simulink model "inverseDynamicsControl"  (R2023b)
settings: Solver=VariableStepAuto  StartTime=0.0  StopTime=time(end)  RelTol=1e-3
undefined symbols (not defined in the file): DiscIntNeverNeededParam
libraries: simulink x1, slpidlib x1
settings Model: Creator=v4pal  LastModifiedBy=v4pal

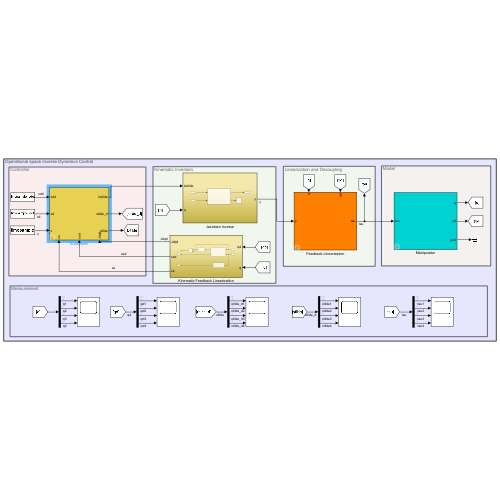
[thumbnail: Simulink's stored preview of the top-level diagram]
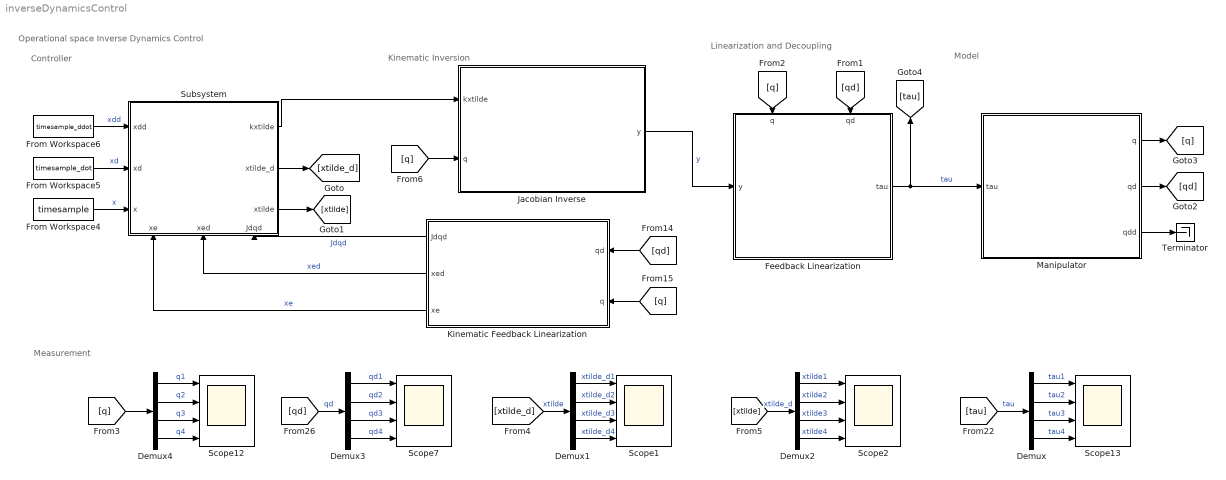
== system inverseDynamicsControl ==
  note: Measurement
  note: Operational space Inverse Dynamics Control
  note: Controller
  note: Kinematic Inversion
  note: Model
  note: Linearization and Decoupling
  Demux{,1..4} (5 alike) : Demux
  Feedback Linearization : Subsystem  mask{m_load=4}
      mask prompts: m_load "Load Mass [kg]"
      settings: PortSchema="{\"entries\":[{\"content\":{\"sides\":[{\"content\":{\"connectorIds\":[\"In1\"]},\"type\":\"ConnectorPlacement.EquallySpacedRectSide\",\"uuid\":\"271cc0a6-b732-4626-ad15-944ba501bea2\"},{\"content\":{\"connectorIds\":[\"Out1\"],\"side\":\"RIGHT\"},\"type\":\"ConnectorPlacement.EquallySpacedRectSide\",\"uuid\":\"860ec51b-c9e7-4b7b-ae65-2fc3300d48f6\"},{\"content\":{\"connectorIds\":[\"In2\",\"In3\"],\"side\":\"TOP\"},\"type\":\"ConnectorPlacement.EquallySpacedRectSide\",\"uuid\":\"a378ade9-13de-47ec-a220-3e435cc4dc56\"},{\"content\":{\"side\":\"BOTTOM\"},\"type\":\"ConnectorPlacement.EquallySpacedRectSide\",\"uuid\":\"8c63b252-3c1f-48d2-9139-67a3c74d1549\"}]},\"type\":\"ConnectorPlacement.EquallySpacedConnector\",\"uuid\":\"fa57dee9-db69-4719-bb64-b991f88f74fb\"}],\"packageUris\":[\"http://schema.mathworks.com/mf0/Connector/R2020b\"],\"version\":\"1.0\"}"
      mask DialogControl DescGroupVar Prompt: Nonlinear Compensation
      mask DialogControl DescTextVar Prompt: Nonlinear compensation and decoupling block
  From Workspace4 : FromWorkspace  VariableName=timesample
  From Workspace5 : FromWorkspace  VariableName=timesample_dot
  From Workspace6 : FromWorkspace  VariableName=timesample_ddot
  Jacobian Inverse : Subsystem
  Kinematic Feedback Linearization : Subsystem
  Manipulator : Subsystem  mask{m_load=4, delta=0.0}
      mask prompts: m_load "Load Mass [kg]"; delta "Uncertainty [%]"
      mask DialogControl DescGroupVar Prompt: SCARA Dynamic Model
      mask DialogControl DescTextVar Prompt: Scara Dynamic Model with uncertainty and load mass as input.
  Scope{1..2,7,12..13} (5 alike) : Scope  NumInputPorts=4
  Subsystem : Subsystem  mask{Kd=15, Kp=150, Ki=0}
      settings: PortSchema="{\"entries\":[{\"content\":{\"sides\":[{\"content\":{\"connectorIds\":[\"In1\",\"In2\",\"In3\"]},\"type\":\"ConnectorPlacement.EquallySpacedRectSide\",\"uuid\":\"d5d0fa15-0dfc-4de5-8b58-3094a24c3543\"},{\"content\":{\"connectorIds\":[\"Out1\",\"Out2\",\"Out3\"],\"side\":\"RIGHT\"},\"type\":\"ConnectorPlacement.EquallySpacedRectSide\",\"uuid\":\"dc48d10e-f543-4bb1-aabf-9e7d159af175\"},{\"content\":{\"side\":\"TOP\"},\"type\":\"ConnectorPlacement.EquallySpacedRectSide\",\"uuid\":\"cd48e311-8a6b-415c-be96-943e62210695\"},{\"content\":{\"connectorIds\":[\"In4\",\"In5\",\"In6\"],\"side\":\"BOTTOM\"},\"type\":\"ConnectorPlacement.EquallySpacedRectSide\",\"uuid\":\"938f084a-ffdf-47d0-9ea2-b90851473a83\"}]},\"type\":\"ConnectorPlacement.EquallySpacedConnector\",\"uuid\":\"fa3c2d25-ad58-4bec-8aba-e67d02255a63\"}],\"packageUris\":[\"http://schema.mathworks.com/mf0/Connector/R2020b\"],\"version\":\"1.0\"}"
  Terminator : Terminator
  wires:
  [qd] -> Kinematic Feedback Linearization/1(qd)
  [q] -> Kinematic Feedback Linearization/2(q)
  Feedback Linearization/1(tau) -> Manipulator/1(tau), [tau]  "tau"
  [qd] -> Feedback Linearization/3(qd)
  [q] -> Feedback Linearization/2(q)
  Manipulator/3(qdd) -> Terminator/1
  From Workspace6/1 -> Subsystem/1(xdd)  "xdd"
  From Workspace5/1 -> Subsystem/2(xd)  "xd"
  From Workspace4/1 -> Subsystem/3(x)  "x"
  Kinematic Feedback Linearization/1(Jdqd) -> Subsystem/6(Jdqd)  "Jdqd"
  Kinematic Feedback Linearization/2(xed) -> Subsystem/5(xed)  "xed"
  Kinematic Feedback Linearization/3(xe) -> Subsystem/4(xe)  "xe"
  Subsystem/1(kxtilde) -> Jacobian Inverse/1(kxtilde)
  Subsystem/2(xtilde_d) -> [xtilde_d]
  Subsystem/3(xtilde) -> [xtilde]
  Demux2/4 -> Scope2/4  "xtilde4"
  Demux2/3 -> Scope2/3  "xtilde3"
  Demux2/2 -> Scope2/2  "xtilde2"
  Demux2/1 -> Scope2/1  "xtilde1"
  Demux/2 -> Scope13/2  "tau2"
  Demux3/1 -> Scope7/1  "qd1"
  Demux1/1 -> Scope1/1  "xtilde_d1"
  Demux/3 -> Scope13/3  "tau3"
  [xtilde_d] -> Demux1/1  "xtilde"
  Demux1/3 -> Scope1/3  "xtilde_d3"
  [q] -> Demux4/1
  Demux3/4 -> Scope7/4  "qd4"
  Demux3/3 -> Scope7/3  "qd3"
  Demux3/2 -> Scope7/2  "qd2"
  Demux1/2 -> Scope1/2  "xtilde_d2"
  Demux1/4 -> Scope1/4  "xtilde_d4"
  [xtilde] -> Demux2/1  "xtilde_d"
  Demux4/2 -> Scope12/2  "q2"
  Demux4/4 -> Scope12/4  "q4"
  [tau] -> Demux/1  "tau"
  Demux/1 -> Scope13/1  "tau1"
  Demux4/3 -> Scope12/3  "q3"
  Demux/4 -> Scope13/4  "tau4"
  Demux4/1 -> Scope12/1  "q1"
  [qd] -> Demux3/1  "qd"
  Jacobian Inverse/1(y) -> Feedback Linearization/1(y)  "y"
  [q] -> Jacobian Inverse/2(q)
  Manipulator/1(q) -> [q]
  Manipulator/2(qd) -> [qd]

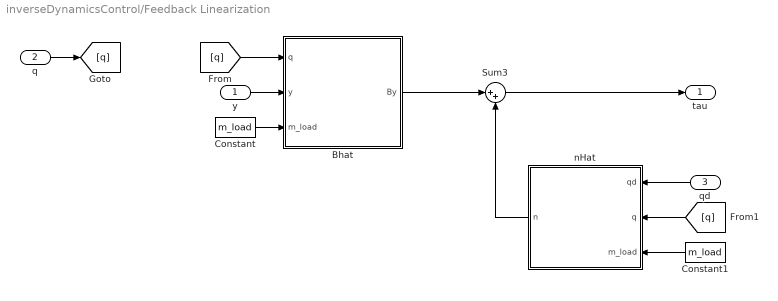
== system inverseDynamicsControl/Feedback Linearization ==
  y : Inport
  q : Inport  Port=2
  qd : Inport  Port=3
  Bhat : MATLAB Function  TreatAsAtomicUnit=on
  Constant : Constant  Value=m_load
  Constant1 : Constant  Value=m_load
  Sum3 : Sum  Inputs=|++
  nHat : MATLAB Function  TreatAsAtomicUnit=on
  tau : Outport
  wires:
  nHat/1(n) -> Sum3/2
  [q] -> nHat/2(q)
  qd/1 -> nHat/1(qd)
  Sum3/1 -> tau/1
  Bhat/1(By) -> Sum3/1
  y/1 -> Bhat/2(y)
  Constant/1 -> Bhat/3(m_load)
  Constant1/1 -> nHat/3(m_load)
  q/1 -> [q]
  [q] -> Bhat/1(q)

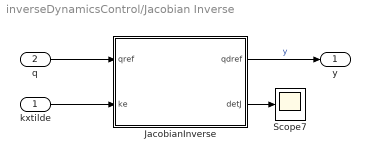
== system inverseDynamicsControl/Jacobian Inverse ==
  kxtilde : Inport
  q : Inport  Port=2
  JacobianInverse : MATLAB Function  TreatAsAtomicUnit=on
  Scope7 : Scope
  y : Outport
  wires:
  JacobianInverse/2(detJ) -> Scope7/1
  JacobianInverse/1(qdref) -> y/1  "y"
  kxtilde/1 -> JacobianInverse/2(ke)
  q/1 -> JacobianInverse/1(qref)

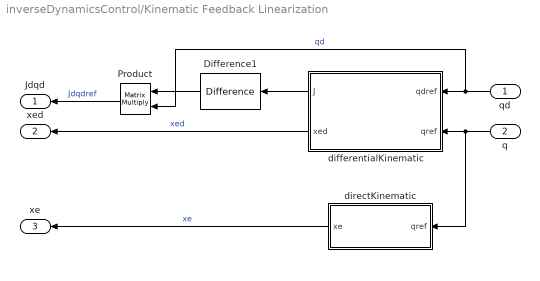
== system inverseDynamicsControl/Kinematic Feedback Linearization ==
  qd : Inport
  q : Inport  Port=2
  Difference1 : simulink/Discrete/Difference  ICPrevInput=0.0  OutMin=[]  OutMax=[]  OutDataType=fixdt(1, 16)  OutScaling=2^-10  DoSatur=off
  Product : Product  Multiplication=Matrix(*)
  differentialKinematic : MATLAB Function  TreatAsAtomicUnit=on
  directKinematic : MATLAB Function  TreatAsAtomicUnit=on
  Jdqd : Outport
  xed : Outport  Port=2
  xe : Outport  Port=3
  wires:
  Product/1 -> Jdqd/1  "Jdqdref"
  Difference1/1 -> Product/1
  q/1 -> directKinematic/1(qref), differentialKinematic/2(qref)
  differentialKinematic/2(xed) -> xed/1  "xed"
  qd/1 -> Product/2, differentialKinematic/1(qdref)  "qd"
  differentialKinematic/1(J) -> Difference1/1
  directKinematic/1(xe) -> xe/1  "xe"

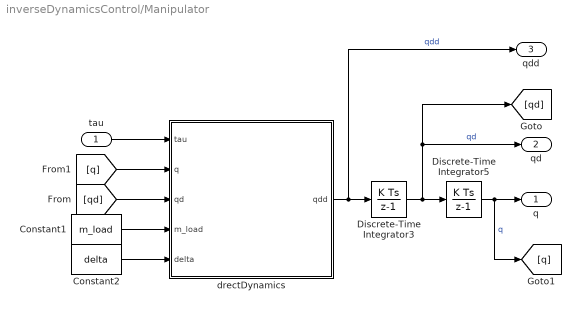
== system inverseDynamicsControl/Manipulator ==
  tau : Inport
  Constant1 : Constant  Value=m_load
  Constant2 : Constant  Value=delta
  Discrete-Time Integrator3 : DiscreteIntegrator  InitialCondition=[0; 0; 0; 0]  SampleTime=0.001  ICPrevOutput=DiscIntNeverNeededParam  ICPrevScaledInput=DiscIntNeverNeededParam
  Discrete-Time Integrator5 : DiscreteIntegrator  InitialCondition=[-1.5706; 0.7851; 0.5000; -0.7855]  SampleTime=0.001  ICPrevOutput=DiscIntNeverNeededParam  ICPrevScaledInput=DiscIntNeverNeededParam
  drectDynamics : MATLAB Function  TreatAsAtomicUnit=on
  q : Outport
  qd : Outport  Port=2
  qdd : Outport  Port=3
  wires:
  tau/1 -> drectDynamics/1(tau)
  Constant1/1 -> drectDynamics/4(m_load)
  drectDynamics/1(qdd) -> qdd/1, Discrete-Time Integrator3/1  "qdd"
  Discrete-Time Integrator3/1 -> [qd], qd/1, Discrete-Time Integrator5/1  "qd"
  Discrete-Time Integrator5/1 -> [q], q/1  "q"
  [qd] -> drectDynamics/3(qd)
  [q] -> drectDynamics/2(q)
  Constant2/1 -> drectDynamics/5(delta)

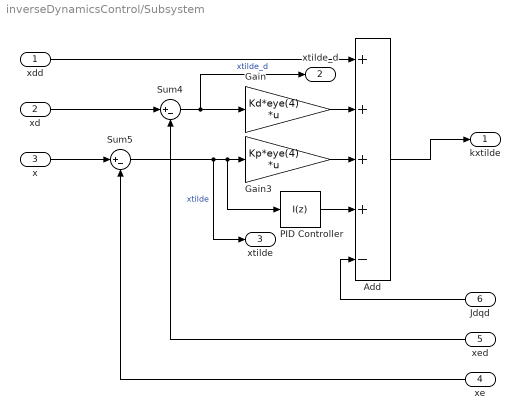
== system inverseDynamicsControl/Subsystem ==
  xdd : Inport
  xd : Inport  Port=2
  x : Inport  Port=3
  xe : Inport  Port=4
  xed : Inport  Port=5
  Jdqd : Inport  Port=6
  Add : Sum  Inputs=++++-
  Gain : Gain  Gain=Kd*eye(4)  Multiplication=Matrix(K*u)
  Gain3 : Gain  Gain=Kp*eye(4)  Multiplication=Matrix(K*u)
  PID Controller : slpidlib/PID Controller  Controller=I  Form=Parallel  TimeDomain=Discrete-time  UseExternalTs=off  SampleTime=-1  IntegratorMethod=Forward Euler  FilterMethod=Forward Euler  ControllerParametersSource=internal  P=1  I=Ki  UseKiTs=off  D=0  N=100  UseFilter=on  TunerSelectOption=Transfer Function Based (PID Tuner App)  InitialConditionSource=internal  InitialConditionForIntegrator=0  InitialConditionForFilter=0  DifferentiatorICPrevScaledInput=0  ExternalReset=none  TrackingMode=off  Kt=1  LimitOutput=off  SatLimitsSource=internal  UpperSaturationLimit=inf  LowerSaturationLimit=-inf  LinearizeAsGain=on  AntiWindupMode=none  Kb=1  LimitIntegrator=off  UpperIntegratorSaturationLimit=inf  LowerIntegratorSaturationLimit=-inf  POutMin=[]  POutMax=[]  IOutMin=[]  IOutMax=[]  DOutMin=[]  DOutMax=[]  NOutMin=[]  NOutMax=[]  SumOutMin=[]  SumOutMax=[]  SaturationOutMin=[]  SaturationOutMax=[]  PParamMin=[]  PParamMax=[]  IParamMin=[]  IParamMax=[]  DParamMin=[]  DParamMax=[]  NParamMin=[]  NParamMax=[]  KbParamMin=[]  KbParamMax=[]  KtParamMin=[]  KtParamMax=[]  KbOutMin=[]  KbOutMax=[]  KtOutMin=[]  KtOutMax=[]  IntegratorOutMin=[]  IntegratorOutMax=[]  FilterOutMin=[]  FilterOutMax=[]  SumI1OutMin=[]  SumI1OutMax=[]  SumI2OutMin=[]  SumI2OutMax=[]  SumI3OutMin=[]  SumI3OutMax=[]  SumI4OutMin=[]  SumI4OutMax=[]  SumDOutMin=[]  SumDOutMax=[]  DifferentiatorOutMin=[]  DifferentiatorOutMax=[]  FilterDiffOutCoefMin=[]  FilterDiffOutCoefMax=[]  ReciprocalOutMin=[]  ReciprocalOutMax=[]  SumDenOutMin=[]  SumDenOutMax=[]  SumNumOutMin=[]  SumNumOutMax=[]  DivideOutMin=[]  DivideOutMax=[]  UdiffTsProdOutMin=[]  UdiffTsProdOutMax=[]  NTsProdOutMin=[]  NTsProdOutMax=[]  UintegralTsProdOutMin=[]  UintegralTsProdOutMax=[]  UngainTsProdOutMin=[]  UngainTsProdOutMax=[]  ClampingZeroOutDataTypeStr=Inherit: Inherit via back propagation  ClampingZeroOutMin=[]  ClampingZeroOutMax=[]  FilterDenConstantOutDataTypeStr=Inherit: Inherit via back propagation  FilterDenConstantOutMin=[]  FilterDenConstantOutMax=[]  PCopyOutDataTypeStr=Inherit: Inherit via back propagation  PCopyOutMin=[]  PCopyOutMax=[]  NCopyOutDataTypeStr=Inherit: Inherit via back propagation  NCopyOutMin=[]  NCopyOutMax=[]  IntegratorContinuousStateAttributes=''  IntegratorStateMustResolveToSignalObject=off  IntegratorRTWStateStorageClass=Auto  FilterContinuousStateAttributes=''  FilterStateMustResolveToSignalObject=off  FilterRTWStateStorageClass=Auto  ParallelPVariant=Disabled  IdealPVariant=Disabled  IVariant=InternalParameters  DVariant=Disabled  IntegratorVariant=Discrete  SatVariant=Disabled  AWVariant=Passthrough  PCopyVariant=Disabled  TRVariant=Disabled  FdbkBlocksVariant=Forward  IdealPFdbkVariant=Disabled  SatFdbkVariant=Disabled  DerivativeFilterVariant=Disabled  NVariant=Disabled  NCopyVariant=Disabled_SignalSpec  FilterICVariant=Disabled  IntegratorICVariant=InternalICs  ExternalResetVariant=Disabled  TRSumVariant=Passthrough  SumFdbkVariant=Disabled  SumVariant=Passthrough_I  TsampFilterVariant=InternalTs  TsampNgainVariant=Passthrough  TsampIntegralVariant=Disabled_SignalSpec  ExternalSaturationOutDataTypeStr=Inherit: Same as second input
  Sum4 : Sum  Inputs=|+-
  Sum5 : Sum  Inputs=|+-
  kxtilde : Outport
  xtilde_d : Outport  Port=2
  xtilde : Outport  Port=3
  wires:
  xd/1 -> Sum4/1
  Sum5/1 -> xtilde/1, PID Controller/1, Gain3/1  "xtilde"
  x/1 -> Sum5/1
  Gain3/1 -> Add/3
  Sum4/1 -> xtilde_d/1, Gain/1  "xtilde_d"
  Add/1 -> kxtilde/1
  Gain/1 -> Add/2
  xed/1 -> Sum4/2
  xdd/1 -> Add/1
  xe/1 -> Sum5/2
  Jdqd/1 -> Add/5
  PID Controller/1 -> Add/4

== matlab function inverseDynamicsControl/Manipulator/drectDynamics ==
  data: tau input; q input; qdd output; qd input; m_load input; delta input
function qdd = directDynamics(tau,q,qd,m_load,delta)

%% Needed joint position and velocity
q1 = q(1,:);
q2 = q(2,:);
q3 = q(3,:);
qd1 = qd(1,:);
qd2 = qd(2,:);

%% Dynamic Parameters
a1 = 0.5; a2 = 0.5; d0 = 1;
ml1 = 20; ml2 = 20; ml3 = 10;
Il1 = 4; Il2 = 4; Il4 = 1;
Im1 = 0.01; Im2 = 0.01; Im3 = 0.005; Im4 = 0.001;
l1 = 0.25; l2 = 0.25;
kr1 = 1; kr2 = 1; kr3 = 50; kr4 = 20;
Fm1 =  0.00005; Fm2 =  0.00005; Fm3 = 0.01; Fm4 = 0.005;

%% Adding Uncertainty
delta = delta/100; % converting from percentage 
ml1 = ml1 + delta*ml1; ml2 = ml2 + delta*ml2; ml3 = ml3 + delta*ml3;
Il1 = Il1 + delta*Il1; Il2 = Il2 + delta*Il2; Il4 = Il4 + delta*Il4;
l1 = l1 + delta*l1; l2 = l2 + delta*l2;
Fm1 = Fm1 + delta*Fm1;


%% Position vector and z unit vector 
p0 = [0 ; 0 ; d0];
p1 = [a1*cos(q1) ; a1*sin(q1) ; d0];
p2 = [a1*cos(q1) + a2*cos(q1+q2) ; a1*sin(q1) + a2*sin(q1+q2) ; d0];
p3 = p2 - [0 ; 0 ; q3];
p4 = p3;
pl1 = [l1*cos(q1) ; l1*sin(q1) ; d0];
pl2 = [a1*cos(q1) + l2*cos(q1+q2) ; a1*sin(q1) + l2*sin(q1+q2) ; d0];
pl3 = p3; % ????
pl4 = p4; % 
z0 = [0 0 1]';
z1 = [0 0 1]';
z2 = [0 0 -1]';
z3 = [0 0 -1]';

%% Positional and orientation jacobian of links (JPl JOl JOm)
JP_l1 = [cross(z0,pl1-p0) zeros(3,3)];
JP_l2 = [cross(z0,pl2-p0) cross(z1,pl2-p1) zeros(3,2)];
JP_l3 = [cross(z0,pl3-p0) cross(z1,pl3-p1) z2 zeros(3,1)]; 
JP_l4 = [cross(z0,pl4-p0) cross(z1,pl4-p1) z2 cross(z3,pl4-p3)]; %m4=mload

JO_l1 = [z0 zeros(3,3)];
JO_l2 = [z0 z1 zeros(3,2)];
%JO_l3 = [z0 z1 zeros(3,2)]; Il3=0
JO_l4 = [z0 z1 zeros(3,1) z3];

%assuming zm1=z0, zm2=z1, zm3=-z2, zm4=z3-->it's on the joint
JO_m1 = JO_l1;
JO_m1(:,1) = kr1*z0;
JO_m2 = JO_l2;  
JO_m2(:,2) = kr2*z1;
JO_m3 = [z0 z1 zeros(3,2)]; 
JO_m3(:,3) = kr3*z2;
JO_m4 = JO_l4;
JO_m4(:,4) = kr4*z3;

%% Inertia matrix B (eq 7.32)
B1 = ml1*(JP_l1'*JP_l1) + Il1*(JO_l1'*JO_l1) + Im1*(JO_m1'*JO_m1) ; 
B2 = ml2*(JP_l2'*JP_l2) + Il2*(JO_l2'*JO_l2) + Im2*(JO_m2'*JO_m2) ; 
B3 = ml3*(JP_l3'*JP_l3) + 0 + Im3*(JO_m3'*JO_m3) ; %Il3=0
B4 = m_load*(JP_l4'*JP_l4) + Il4*(JO_l4'*JO_l4) + Im4*(JO_m4'*JO_m4) ; 
B = B1 + B2 + B3 + B4;

%% Gravity forces(Formula 7.39)
g0 = [0 0 -9.81]';
g1 = - (ml1*g0'*JP_l1(:,1) + ml2*g0'*JP_l2(:,1) + ml3*g0'*JP_l3(:,1) + m_load*g0'*JP_l4(:,1));
g2 = - (ml1*g0'*JP_l1(:,2) + ml2*g0'*JP_l2(:,2) + ml3*g0'*JP_l3(:,2) + m_load*g0'*JP_l4(:,2));
g3 = - (ml1*g0'*JP_l1(:,3) + ml2*g0'*JP_l2(:,3) + ml3*g0'*JP_l3(:,3) + m_load*g0'*JP_l4(:,3));
g4 = - (ml1*g0'*JP_l1(:,4) + ml2*g0'*JP_l2(:,4) + ml3*g0'*JP_l3(:,4) + m_load*g0'*JP_l4(:,4));
g = [g1 g2 g3 g4]';

%% Coriolis matrix C
C = [-a1*qd2*sin(q2)*(a2*m_load + a2*ml3 + l2*ml2), -a1*sin(q2)*(qd1 + qd2)*(a2*m_load + a2*ml3 + l2*ml2), 0, 0;
      a1*qd1*sin(q2)*(a2*m_load + a2*ml3 + l2*ml2),  0, 0, 0;
      0, 0, 0, 0;
      0, 0, 0, 0]; 

%% Friction
Fv = diag([kr1^2*Fm1 kr2^2*Fm2 kr3^2*Fm3 kr4^2*Fm4]);

%% Acceleration computation
qdd = inv(B)*(tau - C*qd -Fv*qd -g);

end

== matlab function inverseDynamicsControl/Kinematic Feedback Linearization/differentialKinematic ==
  data: qdref input; J output; qref input; xed output
function [J, xed] = Jacobian(qdref, qref)

    % Init the SCARA manipulator parameters
    a1 = .5; a2 = .5;
    theta1 = qref(1,:); theta2 = qref(2,:);
    
    %% Geometric Jacobian Matrix
    Ja = [-a1*sin(theta1) - a2*sin(theta1 + theta2), - a2*sin(theta1 + theta2), 0, 0;
        a1*cos(theta1) + a2*cos(theta1 + theta2), a2*cos(theta1 + theta2), 0, 0;
        0, 0, -1, 0;
        1, 1, 0, -1;];

    % Vx = Jx1 * qd1 + Jx2 * qd2 +Jx3 * qd3;
    % Vy = Jy1 * qd1 + Jy2 * qd2 +Jy3 * qd3;
    % Vz = Jz1 * qd1 + Jz2 * qd2 +Jz3 * qd3;
    
    %J = Ja(1:3,1:3);
    J = Ja;

    %% Calculation of xe_dot
    xed = J * qdref;

end

== matlab function inverseDynamicsControl/Feedback Linearization/nHat ==
  data: qd input; q input; n output; m_load input
function n = nHat(qd,q,m_load)
    
    q1 = q(1,:);
    q2 = q(2,:);
    q3 = q(3,:);
    qd1 = qd(1,:);
    qd2 = qd(2,:);
    
    %% parametri
    a1 = 0.5;
    a2 = 0.5;
    d0 = 1;
    
    ml1 = 20;
    ml2 = 20;
    ml3 = 10;
    l1 = 0.25;
    l2 = 0.25;
    kr1 = 1;
    kr2 = 1;
    kr3 = 50;
    kr4 = 20;
    Fm1 =  0.00005;
    Fm2 =  0.00005;
    Fm3 = 0.01;
    Fm4 = 0.005;
    
    %% calcolo p pl z
    p0 = [0 ; 0 ; d0];
    p1 = [a1*cos(q1) ; a1*sin(q1) ; d0];
    p2 = [a1*cos(q1) + a2*cos(q1+q2) ; a1*sin(q1) + a2*sin(q1+q2) ; d0];
    p3 = p2 - [0 ; 0 ; q3];
    p4 = p3;
    pl1 = [l1*cos(q1) ; l1*sin(q1) ; d0];
    pl2 = [a1*cos(q1) + l2*cos(q1+q2) ; a1*sin(q1) + l2*sin(q1+q2) ; d0];
    pl3 = p3; % ????
    pl4 = p4; % 
    z0 = [0 0 1]';
    z1 = [0 0 1]';
    z2 = [0 0 -1]';
    z3 = [0 0 -1]';
    
    %% calcolo JPl JOl JOm
    JP_l1 = [cross(z0,pl1-p0) zeros(3,3)];
    JP_l2 = [cross(z0,pl2-p0) cross(z1,pl2-p1) zeros(3,2)];
    JP_l3 = [cross(z0,pl3-p0) cross(z1,pl3-p1) z2 zeros(3,1)]; 
    JP_l4 = [cross(z0,pl4-p0) cross(z1,pl4-p1) z2 cross(z3,pl4-p3)]; %m4=mload

    %% Contributo di gravità sull'iesimo link.(Formula 7.39)
    g0 = [0 0 -9.81]';
    g1 = - (ml1*g0'*JP_l1(:,1) + ml2*g0'*JP_l2(:,1) + ml3*g0'*JP_l3(:,1) + m_load*g0'*JP_l4(:,1));
    g2 = - (ml1*g0'*JP_l1(:,2) + ml2*g0'*JP_l2(:,2) + ml3*g0'*JP_l3(:,2) + m_load*g0'*JP_l4(:,2));
    g3 = - (ml1*g0'*JP_l1(:,3) + ml2*g0'*JP_l2(:,3) + ml3*g0'*JP_l3(:,3) + m_load*g0'*JP_l4(:,3));
    g4 = - (ml1*g0'*JP_l1(:,4) + ml2*g0'*JP_l2(:,4) + ml3*g0'*JP_l3(:,4) + m_load*g0'*JP_l4(:,4));
    g = [g1 g2 g3 g4]';
    
    %% Contributo di accelerazione C
    C = [-a1*qd2*sin(q2)*(a2*m_load + a2*ml3 + l2*ml2), -a1*sin(q2)*(qd1 + qd2)*(a2*m_load + a2*ml3 + l2*ml2), 0, 0;
          a1*qd1*sin(q2)*(a2*m_load + a2*ml3 + l2*ml2),  0, 0, 0;
          0, 0, 0, 0;
          0, 0, 0, 0]; 
    
    %% Attrito viscoso al manipolatore
    Fv = diag([kr1^2*Fm1 kr2^2*Fm2 kr3^2*Fm3 kr4^2*Fm4]);

    n = C*qd + Fv*qd + g;

end

== matlab function inverseDynamicsControl/Feedback Linearization/Bhat ==
  data: q input; By output; y input; m_load input
function By = Bhat(q,y,m_load)
    
    q1 = q(1,:);
    q2 = q(2,:);
    q3 = q(3,:);
    q4 = q(4,:);
    
    %% parametri
    a1 = 0.5;
    a2 = 0.5;
    d0 = 1;
    
    ml1 = 20;
    ml2 = 20;
    ml3 = 10;
    Il1 = 4;
    Il2 = 4;
    Il4 = 1;
    Im1 = 0.01;
    Im2 = 0.01;
    Im3 = 0.005;
    Im4 = 0.001;
    l1 = 0.25;
    l2 = 0.25;
    kr1 = 1;
    kr2 = 1;
    kr3 = 50;
    kr4 = 20;
    Fm1 =  0.00005;
    Fm2 =  0.00005;
    Fm3 = 0.01;
    Fm4 = 0.005;
    
    %% calcolo p pl z
    p0 = [0 ; 0 ; d0];
    p1 = [a1*cos(q1) ; a1*sin(q1) ; d0];
    p2 = [a1*cos(q1) + a2*cos(q1+q2) ; a1*sin(q1) + a2*sin(q1+q2) ; d0];
    p3 = p2 - [0 ; 0 ; q3];
    p4 = p3;
    pl1 = [l1*cos(q1) ; l1*sin(q1) ; d0];
    pl2 = [a1*cos(q1) + l2*cos(q1+q2) ; a1*sin(q1) + l2*sin(q1+q2) ; d0];
    pl3 = p3; % ????
    pl4 = p4; % 
    z0 = [0 0 1]';
    z1 = [0 0 1]';
    z2 = [0 0 -1]';
    z3 = [0 0 -1]';
    
    %% calcolo JPl JOl JOm
    JP_l1 = [cross(z0,pl1-p0) zeros(3,3)];
    JP_l2 = [cross(z0,pl2-p0) cross(z1,pl2-p1) zeros(3,2)];
    JP_l3 = [cross(z0,pl3-p0) cross(z1,pl3-p1) z2 zeros(3,1)]; 
    JP_l4 = [cross(z0,pl4-p0) cross(z1,pl4-p1) z2 cross(z3,pl4-p3)]; %m4=mload
    
    JO_l1 = [z0 zeros(3,3)];
    JO_l2 = [z0 z1 zeros(3,2)];
    %JO_l3 = [z0 z1 zeros(3,2)]; Il3=0
    JO_l4 = [z0 z1 zeros(3,1) z3];
    
    %assumo che zm1=z0, zm2=z1, zm3=-z2, zm4=z3-->si trova sul giunto
    JO_m1 = JO_l1;
    JO_m1(:,1) = kr1*z0;
    JO_m2 = JO_l2;  
    JO_m2(:,2) = kr2*z1;
    JO_m3 = [z0 z1 zeros(3,2)]; 
    JO_m3(:,3) = kr3*z2;
    JO_m4 = JO_l4;
    JO_m4(:,4) = kr4*z3;
    
    %% Matrice d'Inerzia B (eq 7.32)
    B1 = ml1*(JP_l1'*JP_l1) + Il1*(JO_l1'*JO_l1) + Im1*(JO_m1'*JO_m1) ; 
    B2 = ml2*(JP_l2'*JP_l2) + Il2*(JO_l2'*JO_l2) + Im2*(JO_m2'*JO_m2) ; 
    B3 = ml3*(JP_l3'*JP_l3) + 0 + Im3*(JO_m3'*JO_m3) ; %Il3=0
    B4 = m_load*(JP_l4'*JP_l4) + Il4*(JO_l4'*JO_l4) + Im4*(JO_m4'*JO_m4) ; 
    B = B1 + B2 + B3 + B4;
    
    By = B * y;

end

== matlab function inverseDynamicsControl/Kinematic Feedback Linearization/directKinematic ==
  data: qref input; xe output
function xe = directKinematic(qref)
    
    %% Init the SCARA manipulator parameters and Joint variables
    a1 = .5; a2 = .5; d0 = 1;
    theta1 = qref(1,:); theta2 = qref(2,:); d3 = qref(3,:); theta4 = qref(4,:);

    %% Forward Kinematics link for the SCARA
    k = [a1*cos(theta1) + a2*cos(theta1 + theta2);
        a1*sin(theta1) + a2*sin(theta1 + theta2);
        d0 - d3;
        theta1 + theta2 - theta4;];

    xe = k;

end

== matlab function inverseDynamicsControl/Jacobian Inverse/JacobianInverse ==
  data: qref input; ke input; qdref output; detJ output
function [qdref, detJ] = inverseJacobian(qref, ke) % q = [theta1; theta2]

    % Init the SCARA manipulator parameters
    a1 = .5; a2 = .5;

    theta1 = qref(1,:); theta2 = qref(2,:);
    %% Geometric Jacobian Matrix
    J = [-a1*sin(theta1) - a2*sin(theta1 + theta2), - a2*sin(theta1 + theta2), 0, 0;
        a1*cos(theta1) + a2*cos(theta1 + theta2), a2*cos(theta1 + theta2), 0, 0;
        0, 0, -1, 0;
        1, 1, 0, -1;];

    % Vx = Jx1 * qd1 + Jx2 * qd2 +Jx3 * qd3;
    % Vy = Jy1 * qd1 + Jy2 * qd2 +Jy3 * qd3;
    % Vz = Jz1 * qd1 + Jz2 * qd2 +Jz3 * qd3;
    
    %J = J(1:3,1:3);
    
    detJ = det(J);
    % Calculate the inverse of the Jacobian matrix
    J_inv = inv(J);

    % Calculate joint velocities
    qdref = J_inv * ke;

end
